simulink model "closed_1"  (R2019b)
settings: Solver=ode45  StartTime=0.0  StopTime=1.5  RelTol=1e-5  EnableMultiTasking=on
values from neighbouring files (symbols this model uses):
  A = zeros(4,4)    [closed_loop.m]    (also in closed_loop2.m; main.m; open_loop.m)
  B = [0 ... (first row only)    [closed_loop.m]    (also in closed_loop2.m; main.m = zeros(4,1); open_loop.m = zeros(4))
  C = [1  0  0  0 ... (first row only)    [closed_loop.m]    (also in closed_loop2.m; main.m = zeros(4,4); open_loop.m = [1 0 0 0)
  x_d = [theta_desired 0 0 0]    [closed_loop.m]    (also in closed_loop2.m)
undefined symbols (not defined in the file or in its folder): K
settings Model: Creator=magudelo  LastModifiedBy=LouisDecloedt
settings DataIOCC: LimitDataPoints=on  SaveFormat=Array  SignalLoggingSaveFormat=ModelDataLogs  ReturnWorkspaceOutputs=off
settings OptimizationCC: ExpressionDepthLimit=2147483647  LifeSpan=inf
settings DebuggingCC: UnderspecifiedInitializationDetection=Classic  MergeDetectMultiDrivingBlocksExec=none  SolverPrmCheckMsg=warning  FcnCallInpInsideContextMsg=warning  AllowSymbolicDim=off  StateNameClashWarn=warning  SFUnexpectedBacktrackingDiag=warning  SFNoUnconditionalDefaultTransitionDiag=warning  SFExecutionAtInitializationDiag=none  ArithmeticOperatorsInVariantConditions=warning
settings HardwareCC: ProdBitPerPointer=32  ProdBitPerSizeT=32  ProdBitPerPtrDiffT=32  ProdLargestAtomicFloat=None  ProdIntDivRoundTo=Undefined  ProdEndianess=Unspecified  ProdWordSize=32  ProdHWDeviceType=32-bit Generic
settings ModelReferenceCC: PropagateSignalLabelsOutOfModel=off
settings SFSimCC: SimUseLocalCustomCode=off  CustomCodeUndefinedFunction=UseInterfaceOnly
settings RTWCC: RTWUseLocalCustomCode=off
settings CodeAppCC: StateflowObjectComments=on
settings GRTTargetCC: TargetLangStandard=C89/C90 (ANSI)  GeneratePreprocessorConditionals=Disable all  CombineOutputUpdateFcns=off  GRTInterface=on
settings ConfigComp: CovMetricSettings=dw  CovHtmlReporting=on  CovSaveCumulativeToWorkspaceVar=on  CovSaveSingleToWorkspaceVar=on  CovExternalEMLEnable=off

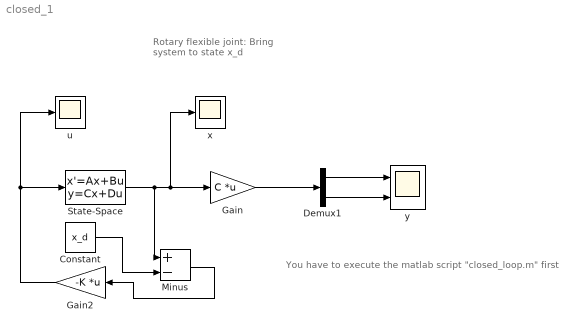
== system closed_1 ==
  note: You have to execute the matlab script "closed_loop.m" first
  note: Rotary flexible joint:
      |  Bring system to state x_d
  Constant : Constant  Value=x_d
  Demux1 : Demux  Outputs=2
  Gain : Gain  Gain=C  Multiplication=Matrix(K*u)
  Gain2 : Gain  Gain=-K  Multiplication=Matrix(K*u)
  Minus : Sum  Inputs=+-
  State-Space : StateSpace  A=A  B=B  C=eye(4)  D=zeros(4,1)  InitialCondition=[0 15*pi/180 0 0]
  u : Scope
  x : Scope
  y : Scope  NumInputPorts=2
  wires:
  State-Space/1 -> x/1, Gain/1, Minus/1
  Gain/1 -> Demux1/1
  Gain2/1 -> u/1, State-Space/1
  Demux1/1 -> y/1
  Demux1/2 -> y/2
  Minus/1 -> Gain2/1
  Constant/1 -> Minus/2
